simulink library "SG_DLE_position_control_module_hose_pump"  (R2025b)
settings: Solver=VariableStepAuto  StartTime=0.0  StopTime=10.0  RelTol=1e-3
undefined symbols (not defined in the file): Ended, IO397, pull, Single, up
libraries: slrealtimeloglib x24, speedgoatlib_IO191 x4, sensor_conversion_blocks x3, simulink x2, DLE_position_controller_v1 x1, DLE_position_controller_v2 x1, speedgoatlib_fpga_analog_io x1, dspstat3 x1, servo_valve_pressure_control_module x1, speedgoatlib_fpga x1
settings Model: Creator=cmmcguir  LastModifiedBy=cmmcguir

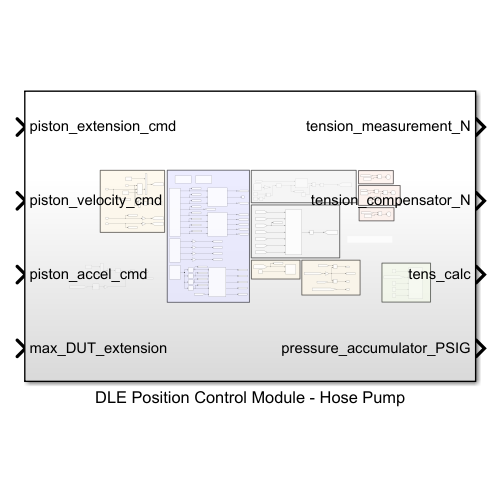
[thumbnail: Simulink's stored preview of the top-level diagram]
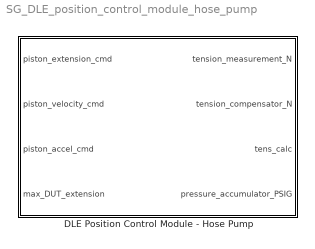
== system SG_DLE_position_control_module_hose_pump ==
  DLE Position Control Module - Hose Pump : Subsystem

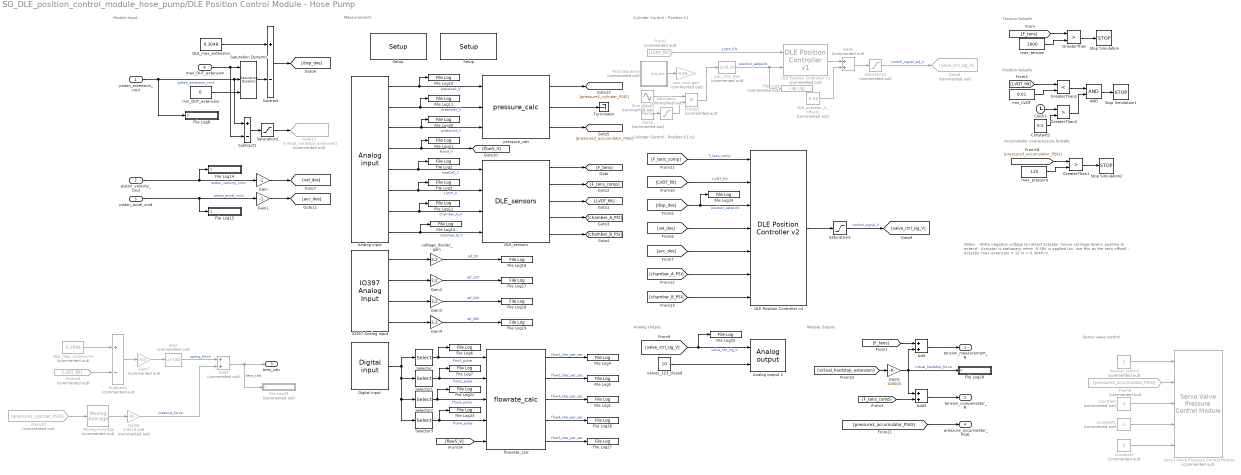
== system SG_DLE_position_control_module_hose_pump/DLE Position Control Module - Hose Pump ==
  note: Analog Output
  note: Measurements
  note: Position failsafe
  note: Tension failsafe
  note: Notes:
      | - Write negative voltage to retract actuator (move carriage down), positive to extend
      | - Actuator is stationary when -0.58V is applied (so, use this as the zero offset)
      | - Actuator max extension = 12 in = 0.3048 m
  note: Cylinder Control - Position CL
  note: Cylinder Control - Position CL v2
  note: Servo valve control
  note: Module Output
  note: Module Input
  note: Accumulator overpressure failsafe
  piston_extension_cmd : Inport
  piston_velocity_cmd : Inport  Port=2
  piston_accel_cmd : Inport  Port=3
  max_DUT_extension : Inport  Port=4
  AND : Logic  AllPortsSameDT=off  OutDataTypeStr=boolean
  Add : Sum
  Add1 : Sum  Commented=on
  Add2 : Sum
  Add4 : Sum  Commented=on
  "Analog input " : speedgoatlib_IO191/Analog input   parModuleId=4  parSampleTime=0.0001  parPciSlot=[12 0]  parAdcChannels=[1 2 3 4 5 6 7 8]  parAdcMode=2  parAdcRanges=[3 3 3 3 3 3 3 3]  parAdcInitValues=[0 0]  parAdcResets=[1 1]  paramsAdcDma=[0 1 200 -1]
      settings: SourceProductName=IO191
  Analog output 2 : speedgoatlib_IO191/Analog output   parModuleId=4  parSampleTime=0.0001  parPciSlot=[12 0]  parDacChannels=[1 2]  parModuleType=1  parDacRanges=[4 4]  parDacInitValues=[0 0]  parDacResets=[1 1]
      settings: SourceProductName=IO191
  Bias : Bias  Commented=on  Bias=185  SaturateOnIntegerOverflow=off
  Clock1 : Clock
  Constant : Constant  Commented=on  Value=-1
  Constant1 : Constant  Commented=on  Value=-1
  Constant2 : Constant  Value=0.5
  Constant3 : Constant  Commented=on  Value=0
  DLE Position Controller v1 : DLE_position_controller_v1/DLE Position Controller v1  Commented=on  SystemSampleTime=-1  VariantActivationTime=update diagram  EmptyChoice=off  PassThrough=off  PassThroughVariantControl=(default)  EmptyChoiceVariantControl=(default)  AllowFlexibleInterface=on  Latency=0  AutoFrameSizeCalculation=off
  DLE Position Controller v2 : DLE_position_controller_v2/DLE Position Controller v2  SystemSampleTime=-1  VariantActivationTime=update diagram  EmptyChoice=off  PassThrough=off  PassThroughVariantControl=(default)  EmptyChoiceVariantControl=(default)  AllowFlexibleInterface=on  Latency=0  AutoFrameSizeCalculation=off
  DLE_actuator_V_offset1 : Constant  Commented=on  Value=-0.58
  DLE_max_extension : Constant  Value=0.3048
  DLE_max_extension1 : Constant  Commented=on  Value=0.3048
  DLE_sensors : sensor_conversion_blocks/DLE_sensors  SystemSampleTime=-1  VariantActivationTime=update diagram  EmptyChoice=off  PassThrough=off  PassThroughVariantControl=(default)  EmptyChoiceVariantControl=(default)  AllowFlexibleInterface=on  Latency=0  AutoFrameSizeCalculation=off
  "Digital input " : speedgoatlib_IO191/Digital input   parModuleId=4  parSampleTime=0.0001  parPortConf=1 port with a 16 elements vector  parDataType=Boolean  parPciSlot=[12 0]  parDiChannels=[1 2 3 4 5 6 7 8]
      settings: SourceProductName=IO191
  File Log{1..7,10..13,16..27} (23 alike) : slrealtimeloglib/File Log  decimation=1  inputProcessing=Elements as channels (sample based)
  File Log14 : Subsystem  mask(slrealtimeloggingblock){decimation=1, inputProcessing=Elements as channels (sample based)}
      mask prompts: decimation "slrealtime:maskStrings:Decimation"; inputProcessing "slrealtime:maskStrings:InputProcessing"
      mask help: slrealtime:maskStrings:FileLogDesc
      mask init:
      | slrealtime.internal.logging.mloggingblock(gcb, decimation, inputProcessing);
      mask Help: eval('slrealtimedoc(''File_Log'')');
      mask TypeOptions inputProcessing: slrealtime:maskStrings:FrameBased | slrealtime:maskStrings:SampleBased
      mask DialogControl DescGroupVar Prompt: File Log
      mask DialogControl decimation Prompt: Decimation
      mask DialogControl inputProcessing Prompt: Input Processing
      mask Display: fprintf(message('slrealtime:maskStrings:FileLogDisp').getString);
  File Log15 : Subsystem  mask(slrealtimeloggingblock){decimation=1, inputProcessing=Elements as channels (sample based)}
      mask prompts: decimation "slrealtime:maskStrings:Decimation"; inputProcessing "slrealtime:maskStrings:InputProcessing"
      mask help: slrealtime:maskStrings:FileLogDesc
      mask init:
      | slrealtime.internal.logging.mloggingblock(gcb, decimation, inputProcessing);
      mask Help: eval('slrealtimedoc(''File_Log'')');
      mask TypeOptions inputProcessing: slrealtime:maskStrings:FrameBased | slrealtime:maskStrings:SampleBased
      mask DialogControl DescGroupVar Prompt: File Log
      mask DialogControl decimation Prompt: Decimation
      mask DialogControl inputProcessing Prompt: Input Processing
      mask Display: fprintf(message('slrealtime:maskStrings:FileLogDisp').getString);
  File Log28 : Subsystem  mask(slrealtimeloggingblock){decimation=1, inputProcessing=Elements as channels (sample based)}
      mask prompts: decimation "slrealtime:maskStrings:Decimation"; inputProcessing "slrealtime:maskStrings:InputProcessing"
      mask help: slrealtime:maskStrings:FileLogDesc
      mask init:
      | slrealtime.internal.logging.mloggingblock(gcb, decimation, inputProcessing);
      mask Help: eval('slrealtimedoc(''File_Log'')');
      mask TypeOptions inputProcessing: slrealtime:maskStrings:FrameBased | slrealtime:maskStrings:SampleBased
      mask DialogControl DescGroupVar Prompt: File Log
      mask DialogControl decimation Prompt: Decimation
      mask DialogControl inputProcessing Prompt: Input Processing
      mask Display: fprintf(message('slrealtime:maskStrings:FileLogDisp').getString);
  File Log29 : Subsystem  Commented=on  mask(slrealtimeloggingblock){decimation=1, inputProcessing=Elements as channels (sample based)}
      mask prompts: decimation "slrealtime:maskStrings:Decimation"; inputProcessing "slrealtime:maskStrings:InputProcessing"
      mask help: slrealtime:maskStrings:FileLogDesc
      mask init:
      | slrealtime.internal.logging.mloggingblock(gcb, decimation, inputProcessing);
      mask Help: eval('slrealtimedoc(''File_Log'')');
      mask TypeOptions inputProcessing: slrealtime:maskStrings:FrameBased | slrealtime:maskStrings:SampleBased
      mask DialogControl DescGroupVar Prompt: File Log
      mask DialogControl decimation Prompt: Decimation
      mask DialogControl inputProcessing Prompt: Input Processing
      mask Display: fprintf(message('slrealtime:maskStrings:FileLogDisp').getString);
  File Log8 : Subsystem  mask(slrealtimeloggingblock){decimation=1, inputProcessing=Elements as channels (sample based)}
      mask prompts: decimation "slrealtime:maskStrings:Decimation"; inputProcessing "slrealtime:maskStrings:InputProcessing"
      mask help: slrealtime:maskStrings:FileLogDesc
      mask init:
      | slrealtime.internal.logging.mloggingblock(gcb, decimation, inputProcessing);
      mask Help: eval('slrealtimedoc(''File_Log'')');
      mask TypeOptions inputProcessing: slrealtime:maskStrings:FrameBased | slrealtime:maskStrings:SampleBased
      mask DialogControl DescGroupVar Prompt: File Log
      mask DialogControl decimation Prompt: Decimation
      mask DialogControl inputProcessing Prompt: Input Processing
      mask Display: fprintf(message('slrealtime:maskStrings:FileLogDisp').getString);
  File Log9 : slrealtimeloglib/File Log  Commented=on  decimation=1  inputProcessing=Elements as channels (sample based)
  From19 : From  Commented=on  GotoTag=LVDT_filt
  From2 : From  Commented=on  GotoTag=LVDT_filt
  From20 : From  Commented=on  GotoTag=pressure1_cylinder_PSIG
  From8 : From  Commented=on  GotoTag=pressure3_accumulator_PSIG
  Gain : Gain  Gain=-1
  Gain1 : Gain  Gain=-1
  Gain2 : Gain  Gain=3.2
  Gain3 : Gain  Gain=3.2
  Gain4 : Gain  Gain=3.2
  Gain5 : Gain  Gain=100000
  Gain7 : Gain  Commented=on  Gain=2626
  Gain8 : Gain  Commented=on  Gain=0.81*4.448
  Goto12 : Goto  Commented=on  GotoTag=virtual_hardstop_extension
  Goto8 : Goto  Commented=on  GotoTag=valve_ctrl_sig_V
  GreaterThan : RelationalOperator  Operator=>  OutDataTypeStr=boolean  RndMeth=Simplest  InputSameDT=off
  GreaterThan1 : RelationalOperator  Operator=>  OutDataTypeStr=boolean  RndMeth=Simplest  InputSameDT=off
  GreaterThan2 : RelationalOperator  Operator=<  OutDataTypeStr=boolean  RndMeth=Simplest  InputSameDT=off
  GreaterThan3 : RelationalOperator  Operator=>  OutDataTypeStr=boolean  RndMeth=Simplest  InputSameDT=off
  IO397 Analog Input : speedgoatlib_fpga_analog_io/IO397/IO397 Analog Input  openMaskCallback=0  id=3  chan=[1 2 3 4]  range=+-10 V  parAiTriggerMode=I/O Module Clock  parAiInternalSignal=None  parAiDioTriggerChannel=1  parAiSampleRate=0  trigger=Initiator  ts=0.0001
      settings: SourceProductName=Analog IO
  Moving Average : dspstat3/Moving Average  Commented=on  Method=Sliding window  ForgettingFactorPort=off  SpecifyWindowLength=on  WindowLength=10  OverlapLength=9  AllowArbitraryInputLength=off  ForgettingFactor=0.9  SimulateUsing=Interpreted execution
  Product : Product  Commented=on
  Ramp : simulink/Sources/Ramp  Commented=on  slope=1/10  start=10  InitialOutput=0
  Saturation : Saturate  Commented=on  UpperLimit=1  LowerLimit=0
  Saturation Dynamic : simulink/Discontinuities/Saturation Dynamic  OutMin=[]  OutMax=[]  OutDataTypeStr=Inherit: Same as second input  OutDataType=fixdt(1, 16)  OutScaling=2^-10  DoSatur=off
  Saturation1 : Saturate  Commented=on  UpperLimit=10  LowerLimit=-10
  Saturation2 : Saturate  UpperLimit=inf  LowerLimit=0
  Saturation5 : Saturate  UpperLimit=10  LowerLimit=-10
  Selector : Selector  InputPortWidth=16  IndexOptions=Index vector (dialog)  Indices=1  OutputSizes=1
  Selector1 : Selector  InputPortWidth=16  IndexOptions=Index vector (dialog)  Indices=2  OutputSizes=1
  Selector2 : Selector  InputPortWidth=16  IndexOptions=Index vector (dialog)  Indices=3  OutputSizes=1
  Selector3 : Selector  InputPortWidth=16  IndexOptions=Index vector (dialog)  Indices=4  OutputSizes=1
  Servo Valve Pressure Control Module : servo_valve_pressure_control_module/Servo Valve Pressure Control Module  Commented=on  SystemSampleTime=-1  VariantActivationTime=update diagram  EmptyChoice=off  PassThrough=off  PassThroughVariantControl=(default)  EmptyChoiceVariantControl=(default)  AllowFlexibleInterface=on  Latency=0  AutoFrameSizeCalculation=off
  Setup : speedgoatlib_fpga/Setup/Setup  Parameter124={}  board=IO397-50k  id=3  pciSlot=-1  device_id=1  bitstreamFilePath=C:\Users\cmmcguir\OneDrive - North Carolina State University\iSSRL\Research\variable-stiffness-WEC\wave_tank_testing\software\speedgoat_IO397_50k_all_io_2\  bitstreamFile=speedgoat_IO397_50k_all_io_2.mat  rearEnb_1=off  rearIO_1=None  rearEnb_2=off  rearIO_2=None  ProgSpiFlash=off  ProgBPIFlash=off  useFpgaDmaController=off  PullRPort15=pull-up 3.3V  PullRPort31=pull-up 3.3V  PullRPort47=pull-up 3.3V  PullRPort63=pull-up 3.3V  diffLineTermination_1=on  diffLineTermination_2=on  diffLineTermination_3=on  diffLineTermination_4=on  diffLineTermination_5=on  diffLineTermination_6=on  diffLineTermination_7=on  diffLineTermination_8=on  diffLineTermination_9=on  diffLineTermination_10=on  diffLineTermination_11=on  diffLineTermination_12=on  diffLineTermination_13=on  diffLineTermination_14=on  diffLineTermination_15=on  diffLineTermination_16=on  diffLineTermination_17=on  diffLineTermination_18=on  diffLineTermination_19=on  diffLineTermination_20=on  diffLineTermination_21=on  diffLineTermination_22=on  diffLineTermination_23=on  diffLineTermination_24=on  diffLineTermination_25=on  diffLineTermination_26=on  diffLineTermination_27=on  diffLineTermination_28=on  diffLineTermination_29=on  diffLineTermination_30=on  diffLineTermination_31=on  diffLineTermination_32=on  Vi_Pull_36x_1=Floating  Vo_36x_1=3.3V  Vi_Pull_36x_2=Floating  Vo_36x_2=3.3V  Vi_Pull_36x_3=Floating  Vo_36x_3=3.3V  Vi_Pull_36x_4=Floating  Vo_36x_4=3.3V  Vi_Pull_36x_5=Floating  Vo_36x_5=3.3V  Vi_Pull_36x_6=Floating  Vo_36x_6=3.3V  Vi_Pull_36x_7=Floating  Vo_36x_7=3.3V  Vi_Pull_36x_8=Floating  Vo_36x_8=3.3V  Vi_Pull_36x_9_16=Floating  Vo_36x_9_16=3.3V  Vi_Pull_36x_17_24=Floating  Vo_36x_17_24=3.3V  Vi_Pull_36x_25_32=Floating  Vo_36x_25_32=3.3V  Vi_Pull_36x_33_40=Floating  Vo_36x_33_40=3.3V  Vi_Pull_36x_41_48=Floating  Vo_36x_41_48=3.3V  Vi_Pull_36x_49_56=Floating  Vo_36x_49_56=3.3V  Vi_Pull_36x_57_64=Floating  Vo_36x_57_64=3.3V  PullRPort0_1=pull-up  VioPort0_1=3.3V  PullRPort1_1=pull-up  VioPort1_1=3.3V  PullRPort2_1=pull-up  VioPort2_1=3.3V  PullRPort3_1=pull-up  VioPort3_1=3.3V  PullRPort4_1=pull-up  VioPort4_1=3.3V  PullRPort5_1=pull-up  VioPort5_1=3.3V  PullRPort6_1=pull-up  VioPort6_1=3.3V  diffLineTermination_rear1_1=on  diffLineTermination_rear1_2=on  diffLineTermination_rear1_3=on  diffLineTermination_rear1_4=on  diffLineTermination_rear1_5=on  diffLineTermination_rear1_6=on  diffLineTermination_rear1_7=on  diffLineTermination_rear1_8=on  PullRPort0_2=pull-up  VioPort0_2=3.3V  PullRPort1_2=pull-up  VioPort1_2=3.3V  PullRPort2_2=pull-up  VioPort2_2=3.3V  PullRPort3_2=pull-up  VioPort3_2=3.3V  PullRPort4_2=pull-up  VioPort4_2=3.3V  PullRPort5_2=pull-up  VioPort5_2=3.3V  PullRPort6_2=pull-up  VioPort6_2=3.3V  diffLineTermination_rear2_1=on  diffLineTermination_rear2_2=on  diffLineTermination_rear2_3=on  diffLineTermination_rear2_4=on  diffLineTermination_rear2_5=on  diffLineTermination_rear2_6=on  diffLineTermination_rear2_7=on  diffLineTermination_rear2_8=on
      settings: SourceProductName=IO3xx
  "Setup " : speedgoatlib_IO191/Setup   parModuleId=4  parPciSlot=[12,0]  parTriggerSignal=TTL  parAdcChannels=[1 2 3 4 5 6 7 8]  parAdcRanges=[3 3 3 3 3 3 3 3]  parAdcChannel1=on  parAdcChannel2=on  parAdcChannel3=on  parAdcChannel4=on  parAdcChannel5=on  parAdcChannel6=on  parAdcChannel7=on  parAdcChannel8=on  parAdcMode=Single-Ended  parAdcRange11=+-10.24 V  parAdcRange21=+-24.576 V  parAdcRange12=+-10.24 V  parAdcRange22=+-24.576 V  parAdcRange13=+-10.24 V  parAdcRange23=+-24.576 V  parAdcRange14=+-10.24 V  parAdcRange24=+-24.576 V  parAdcRange15=+-10.24 V  parAdcRange25=+-24.576 V  parAdcRange16=+-10.24 V  parAdcRange26=+-24.576 V  parAdcRange17=+-10.24 V  parAdcRange27=+-24.576 V  parAdcRange18=+-10.24 V  parAdcRange28=+-24.576 V  parAdcEnDma=off  parAdcFrame=125  parAdcDiv=200  parAdcSample=-1  parDacChannels=[1 2]  parDacChannel1=on  parDacChannel2=on  parDacChannel3=off  parDacChannel4=off  parDacMode=Single-Ended  parDacRanges=[4 4]  parDacInitValues=[0 0]  parDacResets=[1 1]  parDacRange1=+-10 V  parDacInitValue1=0  parDacReset1=on  parDacRange2=+-10 V  parDacInitValue2=0  parDacReset2=on  parDacRange3=+-10 V  parDacInitValue3=0  parDacReset3=on  parDacRange4=+-10 V  parDacInitValue4=0  parDacReset4=on  parDiChannels=[1 2 3 4 5 6 7 8]  parDoChannels=[9 10 11 12 13 14 15 16]  parDioFirstControl=[2 3 4 5 6 7 8 9]  parDioSecondControl=0  parDioChannel1=In  parExtra1=I  parExtra2=I  parExtra3=I  parDioChannel2=Out  parDioChannel3=Out  parDioChannel4=Out  parDioChannel5=Out  parDioChannel6=Out  parDioChannel7=Out  parDioChannel8=Out  parDioChannel9=Out  parDoInitValues=[0 0 0 0]  parDoResets=[1 1 1 1]  parDoInitValue1=0  parDoReset1=on  parDoInitValue2=0  parDoReset2=on  parDoInitValue3=0  parDoReset3=on  parDoInitValue4=0  parDoReset4=on  parDoInitValue5=0  parDoReset5=on  parDoInitValue6=0  parDoReset6=on  parDoInitValue7=0  parDoReset7=on  parDoInitValue8=0  parDoReset8=on  parDoInitValue9=0  parDoReset9=on  parDoInitValue10=0  parDoReset10=on  parDoInitValue11=0  parDoReset11=on  parDoInitValue12=0  parDoReset12=on  parDoInitValue13=0  parDoReset13=on  parDoInitValue14=0  parDoReset14=on  parDoInitValue15=0  parDoReset15=on  parDoInitValue16=0  parDoReset16=on
      settings: SourceProductName=IO191
  Sine Wave1 : Sin  Commented=on  Amplitude=0.04  Frequency=2*pi/2  SampleTime=0
  Stop Simulation : Stop
  Stop Simulation1 : Stop
  Stop Simulation2 : Stop
  Subtract : Sum  Inputs=+-
  Subtract1 : Sum  Inputs=+-
  Subtract2 : Sum  Commented=on  Inputs=+-
  Terminator : Terminator
  Test Sequence : Test Sequence  Commented=on  TreatAsAtomicUnit=on
  flowrate_calc : sensor_conversion_blocks/flowrate_calc  SystemSampleTime=-1  VariantActivationTime=update diagram  EmptyChoice=off  PassThrough=off  PassThroughVariantControl=(default)  EmptyChoiceVariantControl=(default)  AllowFlexibleInterface=on  Latency=0  AutoFrameSizeCalculation=off
  manual_control : Constant  Commented=on  SampleTime=0.0001
  max_pressure : Constant  Value=120
  max_tension : Constant  Value=1000
  min_DUT_extension : Constant  Value=0
  min_LVDT : Constant  Value=0.01
  pos_sine_bias : Bias  Commented=on  Bias=0.24  SaturateOnIntegerOverflow=off
  pos_sine_gain : Gain  Commented=on  Gain=0.04
  pressure_calc : sensor_conversion_blocks/pressure_calc  SystemSampleTime=-1  VariantActivationTime=update diagram  EmptyChoice=off  PassThrough=off  PassThroughVariantControl=(default)  EmptyChoiceVariantControl=(default)  AllowFlexibleInterface=on  Latency=0  AutoFrameSizeCalculation=off
  valves_123_closed : Constant  Value=10
  voltage_divider_gain : Gain  Gain=3.2
  tension_measurement_N : Outport
  tension_compensator_N : Outport  Port=2
  tens_calc : Outport  Port=3
  pressure_accumulator_PSIG : Outport  Port=4
  wires:
  DLE_sensors/5 -> [chamber_B_PSI]
  Constant/1 -> Servo Valve Pressure Control Module/3
  "Analog input "/2 -> pressure_calc/2, File Log11/1  "pressure2_V"
  manual_control/1 -> Servo Valve Pressure Control Module/1
  pressure_calc/3 -> [pressure3_accumulator_PSIG]
  IO397 Analog Input/4 -> Gain4/1
  Sine Wave1/1 -> Product/1
  "Analog input "/4 -> [flow5_V], File Log21/1  "flow5_V"
  [disp_des] -> DLE Position Controller v2/3, File Log24/1  "position_setpoint"
  Gain4/1 -> File Log19/1  "ref_28V"
  From8/1 -> Servo Valve Pressure Control Module/2
  Constant3/1 -> Servo Valve Pressure Control Module/5
  Product/1 -> pos_sine_bias/1
  Selector/1 -> flowrate_calc/1, File Log6/1  "flow1_pulse"
  [F_tens] -> Add/1
  "Analog input "/1 -> pressure_calc/1, File Log10/1  "pressure1_V"
  min_LVDT/1 -> GreaterThan2/2
  "Analog input "/7 -> DLE_sensors/3, File Log12/1  "chamber_A_V"
  GreaterThan2/1 -> AND/1
  Constant1/1 -> Servo Valve Pressure Control Module/4
  "Analog input "/3 -> pressure_calc/3, File Log20/1  "pressure3_V"
  DLE Position Controller v1/1 -> Add1/1
  pressure_calc/1 -> [pressure1_cylinder_PSIG]
  IO397 Analog Input/3 -> Gain3/1
  DLE_actuator_V_offset1/1 -> Add1/2
  Selector3/1 -> flowrate_calc/4, File Log23/1  "flow4_pulse"
  Test Sequence/1(sine_pos) -> pos_sine_gain/1
  pressure_calc/2 -> Terminator/1
  Ramp/1 -> Saturation/1
  flowrate_calc/2 -> File Log5/1  "flow2_liter_per_sec"
  [valve_ctrl_sig_V] -> File Log25/1, Analog output 2/1  "valve_ctrl_sig_V"
  Gain3/1 -> File Log18/1  "ref_24V"
  [F_tens_comp] -> DLE Position Controller v2/1  "F_tens_comp"
  [LVDT_filt] -> DLE Position Controller v2/2  "LVDT_filt"
  GreaterThan/1 -> Stop Simulation/1
  Selector1/1 -> flowrate_calc/2, File Log7/1  "flow2_pulse"
  [flow5_V] -> flowrate_calc/5
  Saturation/1 -> Product/2
  valves_123_closed/1 -> Analog output 2/2
  [LVDT_filt] -> GreaterThan2/1
  flowrate_calc/5 -> File Log27/1  "flow5_liter_per_sec"
  DLE_sensors/1 -> [F_tens]
  flowrate_calc/4 -> File Log26/1  "flow4_liter_per_sec"
  DLE Position Controller v2/1 -> Saturation5/1
  DLE_sensors/3 -> [LVDT_filt]
  "Analog input "/6 -> DLE_sensors/2, File Log3/1  "LVDT_V"
  DLE_sensors/2 -> [F_tens_comp]
  [F_tens] -> GreaterThan/1
  voltage_divider_gain/1 -> File Log16/1  "ref_5V"
  [chamber_B_PSI] -> DLE Position Controller v2/7
  flowrate_calc/1 -> File Log4/1  "flow1_liter_per_sec"
  Selector2/1 -> flowrate_calc/3, File Log22/1  "flow3_pulse"
  max_tension/1 -> GreaterThan/2
  DLE_sensors/4 -> [chamber_A_PSI]
  Constant2/1 -> GreaterThan3/2
  From2/1 -> DLE Position Controller v1/1  "LVDT_filt"
  "Analog input "/5 -> DLE_sensors/1, File Log2/1  "loadCell_V"
  "Analog input "/8 -> DLE_sensors/4, File Log13/1  "chamber_B_V"
  Saturation5/1 -> [valve_ctrl_sig_V]  "control_signal_V"
  IO397 Analog Input/2 -> Gain2/1
  IO397 Analog Input/1 -> voltage_divider_gain/1
  Clock1/1 -> GreaterThan3/1
  pos_sine_bias/1 -> DLE Position Controller v1/2, File Log9/1  "position_setpoint"
  AND/1 -> Stop Simulation1/1
  "Digital input "/1 -> Selector3/1, Selector2/1, Selector1/1, Selector/1
  [chamber_A_PSI] -> DLE Position Controller v2/6
  Add1/1 -> Saturation1/1
  Saturation1/1 -> Goto8/1  "control_signal_adj_V"
  GreaterThan3/1 -> AND/2
  Gain2/1 -> File Log17/1  "ref_12V"
  flowrate_calc/3 -> File Log1/1  "flow3_liter_per_sec"
  Add2/1 -> tension_compensator_N/1
  piston_extension_cmd/1 -> File Log8/1(S), Subtract1/1, Saturation Dynamic/2  "piston_extension_cmd"
  DLE_max_extension/1 -> Subtract/1
  Subtract/1 -> [disp_des]
  piston_velocity_cmd/1 -> File Log14/1(S), Gain/1  "piston_velocity_cmd"
  piston_accel_cmd/1 -> File Log15/1(S), Gain1/1  "piston_accel_cmd"
  [vel_des] -> DLE Position Controller v2/4
  [acc_des] -> DLE Position Controller v2/5
  Gain/1 -> [vel_des]
  Gain1/1 -> [acc_des]
  Saturation Dynamic/1 -> Subtract/2
  max_DUT_extension/1 -> Saturation Dynamic/1, Subtract1/2
  min_DUT_extension/1 -> Saturation Dynamic/3
  Subtract1/1 -> Saturation2/1
  Saturation2/1 -> Goto12/1
  Add/1 -> tension_measurement_N/1
  [virtual_hardstop_extension] -> Gain5/1
  Gain5/1 -> File Log28/1(S), Add2/1, Add/2  "virtual_hardstop_force"
  [F_tens_comp] -> Add2/2
  [pressure3_accumulator_PSIG] -> GreaterThan1/1
  GreaterThan1/1 -> Stop Simulation2/1
  max_pressure/1 -> GreaterThan1/2
  DLE_max_extension1/1 -> Subtract2/1
  From19/1 -> Subtract2/2
  Subtract2/1 -> Gain7/1
  Gain7/1 -> Bias/1
  Bias/1 -> Add4/1  "spring_force"
  From20/1 -> Moving Average/1
  Gain8/1 -> Add4/2  "pressure_force"
  Add4/1 -> File Log29/1(S), tens_calc/1  "tens_calc"
  Moving Average/1 -> Gain8/1
  [pressure3_accumulator_PSIG] -> pressure_accumulator_PSIG/1

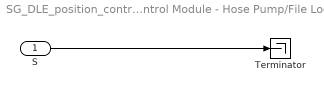
== system SG_DLE_position_control_module_hose_pump/DLE Position Control Module - Hose Pump/File Log14 ==
  S : Inport
  Terminator : Terminator
  wires:
  S/1 -> Terminator/1

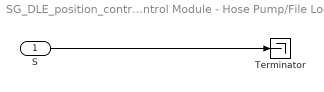
== system SG_DLE_position_control_module_hose_pump/DLE Position Control Module - Hose Pump/File Log15 ==
  S : Inport
  Terminator : Terminator
  wires:
  S/1 -> Terminator/1

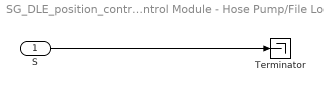
== system SG_DLE_position_control_module_hose_pump/DLE Position Control Module - Hose Pump/File Log28 ==
  S : Inport
  Terminator : Terminator
  wires:
  S/1 -> Terminator/1

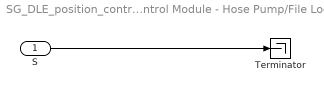
== system SG_DLE_position_control_module_hose_pump/DLE Position Control Module - Hose Pump/File Log29 ==
  S : Inport
  Terminator : Terminator
  wires:
  S/1 -> Terminator/1

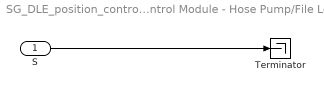
== system SG_DLE_position_control_module_hose_pump/DLE Position Control Module - Hose Pump/File Log8 ==
  S : Inport
  Terminator : Terminator
  wires:
  S/1 -> Terminator/1

== stateflow chart SG_DLE_position_control_module_hose_pump/DLE Position Control Module - Hose Pump/Test Sequence ==
  state step_1
    % apply sine position gain and offset outside of sequence block
    sine_pos = 0;
    % 10 s ramp up, 30 s full, 10 s ramp down --> next sine
  state step_2 % after 10s startup period
    sine_start_timestamp = 10;
    freq = 2*pi / 4; % starting frequency
    sine_t = t - sine_start_timestamp;
    ramp_up_gain = min([1, 1/10*sine_t]);
    ramp_down_gain = min([1, -1/10*sine_t + 5]);
    sine_pos = sin(freq * sine_t) * ramp_up_gain  * ramp_down_gain;
  state step_3
    sine_start_timestamp = 60;
    freq = 2*pi / 3;
    sine_t = t - sine_start_timestamp;
    ramp_up_gain = min([1, 1/10*sine_t]);
    ramp_down_gain = min([1, -1/10*sine_t + 5]);
    sine_pos = sin(freq * sine_t) * ramp_up_gain  * ramp_down_gain;
  state step_4
    sine_start_timestamp = 110;
    freq = 2*pi / 2;
    sine_t = t - sine_start_timestamp;
    ramp_up_gain = min([1, 1/10*sine_t]);
    ramp_down_gain = min([1, -1/10*sine_t + 5]);
    sine_pos = sin(freq * sine_t) * ramp_up_gain  * ramp_down_gain;
  state step_5
    sine_start_timestamp = 160;
    freq = 2*pi / 1;
    sine_t = t - sine_start_timestamp;
    ramp_up_gain = min([1, 1/10*sine_t]);
    ramp_down_gain = min([1, -1/10*sine_t + 5]);
    sine_pos = sin(freq * sine_t) * ramp_up_gain  * ramp_down_gain;
  state step_6
    sine_pos = 0;
  (default) -> step_1
  step_1 -> step_2 % after 10s startup period : [
      | t > 10
      | ]
  step_2 % after 10s startup period -> step_3 : [
      | t > 60
      | ]
  step_3 -> step_4 : [
      | t > 110
      | ]
  step_4 -> step_5 : [
      | t > 160
      | ]
  step_5 -> step_6 : [
      | t > 210
      | ]
  data: sine_pos output; sine_start_timestamp local; freq local; ramp_up_gain local; ramp_down_gain local; sine_t local
